simulink model "mh12_doc"  (Simulink 8.3)
settings: Solver=ode3  StartTime=0.0  StopTime=10  FixedStep=0.01  RelTol=1e-3
values from neighbouring files (symbols this model uses):
  B = [bs1+bs2 -a*bs1+b*bs2 -bs1 -bs2 ... (first row only)    [main1.m]
  K = [ks1+ks2 -a*ks1+b*ks2 -ks1 -ks2 ... (first row only)    [main1.m]
  kt1 = 350000    [main1.m]
  kt2 = 350000    [main1.m]
  M = [ms 0 0 0 ... (first row only)    [main1.m]
settings Model: Creator=thanhcong  LastModifiedBy=HIENANH
settings SolverCC: MaxConsecutiveMinStep=0.1  ZeroCrossControl=DisableAll
settings OptimizationCC: ExpressionDepthLimit=2147483647
settings DebuggingCC: FcnCallInpInsideContextMsg=UseLocalSettings

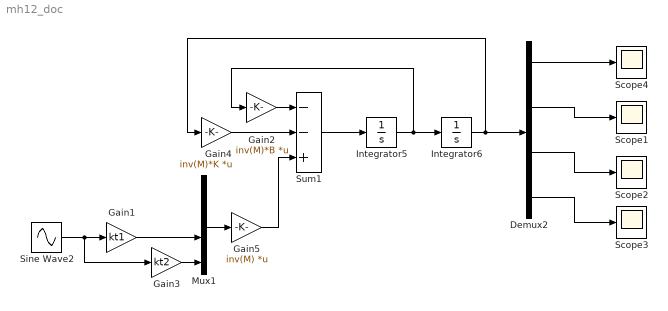
== system mh12_doc ==
  Demux2 : Demux
  Gain1 : Gain  Gain=kt1
  Gain2 : Gain  Gain=inv(M)*B  Multiplication=Matrix(K*u)
  Gain3 : Gain  Gain=kt2
  Gain4 : Gain  Gain=inv(M)*K  Multiplication=Matrix(K*u)
  Gain5 : Gain  Gain=inv(M)  Multiplication=Matrix(K*u)
  Integrator5 : Integrator
  Integrator6 : Integrator
  Mux1 : Mux
  Scope{1..4} (4 alike) : Scope
      Scope2 settings: SaveName=ScopeData2
      Scope3 settings: SaveName=ScopeData3
  Sine Wave2 : Sin  Amplitude=0.05  Frequency=10  SampleTime=0
  Sum1 : Sum  Inputs=--+
  wires:
  Sum1/1 -> Integrator5/1
  Integrator5/1 -> Gain2/1, Integrator6/1
  Gain2/1 -> Sum1/1
  Gain4/1 -> Sum1/2
  Integrator6/1 -> Demux2/1, Gain4/1
  Mux1/1 -> Gain5/1
  Gain5/1 -> Sum1/3
  Sine Wave2/1 -> Gain1/1, Gain3/1
  Demux2/2 -> Scope1/1
  Demux2/3 -> Scope2/1
  Demux2/4 -> Scope3/1
  Gain1/1 -> Mux1/3
  Gain3/1 -> Mux1/4
  Demux2/1 -> Scope4/1
